simulink model "regelung_raum_mdl"  (R2013b)
settings: Solver=ode45  StartTime=0.0  StopTime=7000  MaxStep=0.1  RelTol=1e-3
values from neighbouring files (symbols this model uses):
  Kr = 1 / (K * S)    (= 0.00166666666667)    [wirkungsplan.m]
  Ks = -1 / Kr    (= -600)    [wirkungsplan.m]
  tau = Cp * V / (K * S)    (= 157.5)    [wirkungsplan.m]
libraries: cstblocks x3
settings Model: Creator=daniw  LastModifiedBy=daniw

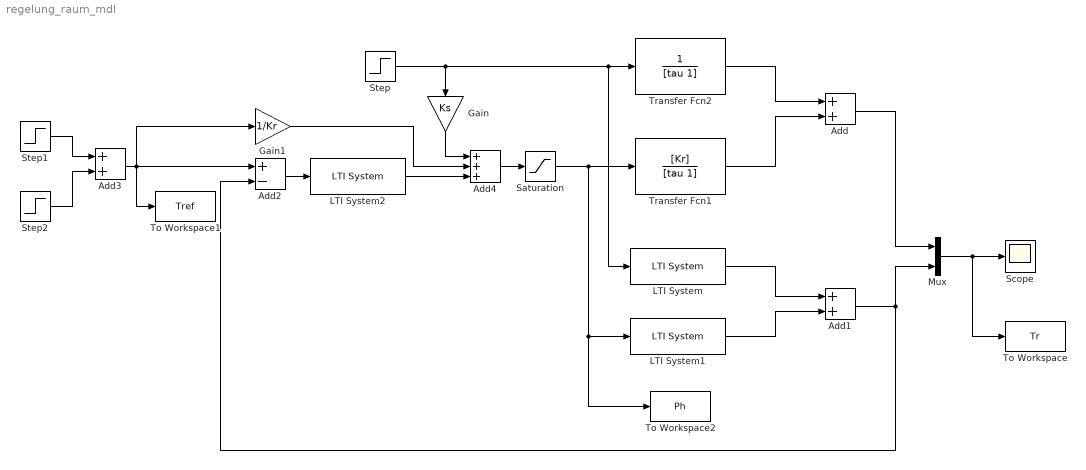
== system regelung_raum_mdl ==
  Add : Sum
  Add1 : Sum
  Add2 : Sum  Inputs=+-
  Add3 : Sum
  Add4 : Sum  Inputs=+++
  Gain : Gain  Gain=Ks
  Gain1 : Gain  Gain=1/Kr
  LTI System : cstblocks/LTI System  sys=G_Tr_Tu  IC=[]
  LTI System1 : cstblocks/LTI System  sys=G_Tr_Ph  IC=[]
  LTI System2 : cstblocks/LTI System  sys=PID_TF  IC=[]
  Mux : Mux  Inputs=2
  Saturation : Saturate  UpperLimit=20e3  LowerLimit=0
  Scope : Scope
  Step : Step  Time=1000  After=-5  SampleTime=0
  Step1 : Step  Time=2500  Before=11  After=20  SampleTime=0
  Step2 : Step  Time=5000  After=-10  SampleTime=0
  To Workspace : ToWorkspace  VariableName=Tr  SampleTime=-1  SaveFormat=Structure With Time
  To Workspace1 : ToWorkspace  VariableName=Tref  SampleTime=-1  SaveFormat=Structure With Time
  To Workspace2 : ToWorkspace  VariableName=Ph  SampleTime=-1  SaveFormat=Structure With Time
  Transfer Fcn1 : TransferFcn  Numerator=[Kr]  Denominator=[tau 1]
  Transfer Fcn2 : TransferFcn  Denominator=[tau 1]
  wires:
  Mux/1 -> To Workspace/1, Scope/1
  Transfer Fcn2/1 -> Add/1
  Transfer Fcn1/1 -> Add/2
  Step/1 -> LTI System/1, Transfer Fcn2/1, Gain/1
  Add3/1 -> Gain1/1, Add2/1, To Workspace1/1
  Add/1 -> Mux/1
  Add1/1 -> Mux/2, Add2/2
  LTI System/1 -> Add1/1
  LTI System1/1 -> Add1/2
  Add2/1 -> LTI System2/1
  Add4/1 -> Saturation/1
  Step1/1 -> Add3/1
  Step2/1 -> Add3/2
  Saturation/1 -> To Workspace2/1, LTI System1/1, Transfer Fcn1/1
  Gain/1 -> Add4/1
  LTI System2/1 -> Add4/3
  Gain1/1 -> Add4/2
